simulink model "CONTROL_SYSTEM_V3_k"  (R2024a)
settings: Solver=ode1  StartTime=0.0  StopTime=inf  FixedStep=0.01  RelTol=1e-5
values from neighbouring files (symbols this model uses):
  Beta1 = 3*Omega_o    (= 15)    [CONTROL_SYSTEM_VAR.m]
  Beta2 = 3*(Omega_o^2)    (= 75)    [CONTROL_SYSTEM_VAR.m]
  Beta3 = (Omega_o^3)    (= 125)    [CONTROL_SYSTEM_VAR.m]
  Desire_Max = 255    [CONTROL_SYSTEM_VAR.m]
  Desire_Min = 0    [CONTROL_SYSTEM_VAR.m]
  Direction_Pin = 1    [CONTROL_SYSTEM_VAR.m]
  EN_Pin = 0    [CONTROL_SYSTEM_VAR.m]
  J_aet = 0.0035    [CONTROL_SYSTEM_VAR.m]
  Kd = 2    [CONTROL_SYSTEM_VAR.m]
  Ki = 4    [CONTROL_SYSTEM_VAR.m]
  Kn = 0.1    [CONTROL_SYSTEM_VAR.m]
  Kp = 1.4    [CONTROL_SYSTEM_VAR.m]
  omga_c = 10    [CONTROL_SYSTEM_VAR.m]
  roa = 0.24    [CONTROL_SYSTEM_VAR.m]
undefined symbols (not defined in the file or in its folder): sigbuilder_block
libraries: arduinolib x30, simulink_extras x14, simulink x5, slpidlib x4, spsOnDelayLib x2, slctrl_autotuning x2, slctrl_adaptive x1
(part 4 of 4)

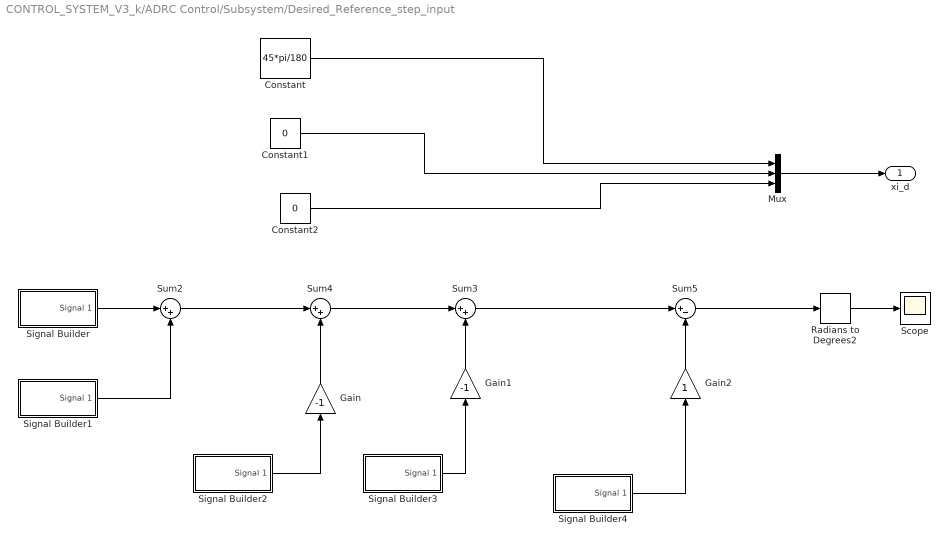
== system CONTROL_SYSTEM_V3_k/ADRC Control/Subsystem/Desired_Reference_step_input ==
  Constant : Constant  Value=45*pi/180
  Constant1 : Constant  Value=0
  Constant2 : Constant  Value=0
  Gain : Gain  Gain=-1
  Gain1 : Gain  Gain=-1
  Gain2 : Gain
  Mux : Mux  Inputs=3
  Radians to Degrees2 : simulink_extras/Transformations/Radians to Degrees
  Scope : Scope
  Signal Builder : Subsystem  Tag=STV Subsys  LoadFcn=sigbuilder_block('load');  StartFcn=sigbuilder_block('start');  StopFcn=sigbuilder_block('stop');  ClipboardFcn=sigbuilder_block('clipboard');  mask(Sigbuilder block){tuvar=[0:10]}
      mask help: Create and generate interchangeable groups of signals whose waveforms are piecewise linear.
      mask init:
      | if ~strcmp(get_param(bdroot(gcbh),'SimulationStatus'),'stopped') tuvar = sigbuilder_block('maskInit'); end
      settings: CopyFcn=sigbuilder_block('copy');  DeleteFcn=sigbuilder_block('delete');  ModelCloseFcn=sigbuilder_block('modelClose');  PreSaveFcn=sigbuilder_block('preSave');  PauseFcn=sigbuilder_block('pause')  ContinueFcn=sigbuilder_block('continue')  NameChangeFcn=sigbuilder_block('namechange');  OpenFcn=sigbuilder_block('open',[437.25 117.75 550.5 394.5 ]);  CloseFcn=sigbuilder_block('close');
      mask Display: plot(0, 0, 100, 100,[2, 2, 32, 32, 2], [68, 8, 8, 68, 68],[32, 2], [38, 38], [32, 19, 2],[53, 60, 44], [32, 17, 17, 2],[16, 16, 31, 31]);txt = getActiveGroup(gcbh);text(2, 100, txt,'verticalAlignment', 'top');
  Signal Builder1 : Subsystem  Tag=STV Subsys  LoadFcn=sigbuilder_block('load');  StartFcn=sigbuilder_block('start');  StopFcn=sigbuilder_block('stop');  ClipboardFcn=sigbuilder_block('clipboard');  mask(Sigbuilder block){tuvar=[0:10]}
      mask help: Create and generate interchangeable groups of signals whose waveforms are piecewise linear.
      mask init:
      | if ~strcmp(get_param(bdroot(gcbh),'SimulationStatus'),'stopped') tuvar = sigbuilder_block('maskInit'); end
      settings: CopyFcn=sigbuilder_block('copy');  DeleteFcn=sigbuilder_block('delete');  ModelCloseFcn=sigbuilder_block('modelClose');  PreSaveFcn=sigbuilder_block('preSave');  PauseFcn=sigbuilder_block('pause')  ContinueFcn=sigbuilder_block('continue')  NameChangeFcn=sigbuilder_block('namechange');  OpenFcn=sigbuilder_block('open',[153 72 550.2 394.8 ]);  CloseFcn=sigbuilder_block('close');
      mask Display: plot(0, 0, 100, 100,[2, 2, 32, 32, 2], [68, 8, 8, 68, 68],[32, 2], [38, 38], [32, 19, 2],[53, 60, 44], [32, 17, 17, 2],[16, 16, 31, 31]);txt = getActiveGroup(gcbh);text(2, 100, txt,'verticalAlignment', 'top');
  Signal Builder2 : Subsystem  Tag=STV Subsys  LoadFcn=sigbuilder_block('load');  StartFcn=sigbuilder_block('start');  StopFcn=sigbuilder_block('stop');  ClipboardFcn=sigbuilder_block('clipboard');  mask(Sigbuilder block){tuvar=[0:10]}
      mask help: Create and generate interchangeable groups of signals whose waveforms are piecewise linear.
      mask init:
      | if ~strcmp(get_param(bdroot(gcbh),'SimulationStatus'),'stopped') tuvar = sigbuilder_block('maskInit'); end
      settings: CopyFcn=sigbuilder_block('copy');  DeleteFcn=sigbuilder_block('delete');  ModelCloseFcn=sigbuilder_block('modelClose');  PreSaveFcn=sigbuilder_block('preSave');  PauseFcn=sigbuilder_block('pause')  ContinueFcn=sigbuilder_block('continue')  NameChangeFcn=sigbuilder_block('namechange');  OpenFcn=sigbuilder_block('open',[437.25 117.75 550.5 394.5 ]);  CloseFcn=sigbuilder_block('close');
      mask Display: plot(0, 0, 100, 100,[2, 2, 32, 32, 2], [68, 8, 8, 68, 68],[32, 2], [38, 38], [32, 19, 2],[53, 60, 44], [32, 17, 17, 2],[16, 16, 31, 31]);txt = getActiveGroup(gcbh);text(2, 100, txt,'verticalAlignment', 'top');
  Signal Builder3 : Subsystem  Tag=STV Subsys  LoadFcn=sigbuilder_block('load');  StartFcn=sigbuilder_block('start');  StopFcn=sigbuilder_block('stop');  ClipboardFcn=sigbuilder_block('clipboard');  mask(Sigbuilder block){tuvar=[0:10]}
      mask help: Create and generate interchangeable groups of signals whose waveforms are piecewise linear.
      mask init:
      | if ~strcmp(get_param(bdroot(gcbh),'SimulationStatus'),'stopped') tuvar = sigbuilder_block('maskInit'); end
      settings: CopyFcn=sigbuilder_block('copy');  DeleteFcn=sigbuilder_block('delete');  ModelCloseFcn=sigbuilder_block('modelClose');  PreSaveFcn=sigbuilder_block('preSave');  PauseFcn=sigbuilder_block('pause')  ContinueFcn=sigbuilder_block('continue')  NameChangeFcn=sigbuilder_block('namechange');  OpenFcn=sigbuilder_block('open',[437.25 117.75 550.5 394.5 ]);  CloseFcn=sigbuilder_block('close');
      mask Display: plot(0, 0, 100, 100,[2, 2, 32, 32, 2], [68, 8, 8, 68, 68],[32, 2], [38, 38], [32, 19, 2],[53, 60, 44], [32, 17, 17, 2],[16, 16, 31, 31]);txt = getActiveGroup(gcbh);text(2, 100, txt,'verticalAlignment', 'top');
  Signal Builder4 : Subsystem  Tag=STV Subsys  LoadFcn=sigbuilder_block('load');  StartFcn=sigbuilder_block('start');  StopFcn=sigbuilder_block('stop');  ClipboardFcn=sigbuilder_block('clipboard');  mask(Sigbuilder block){tuvar=[0:10]}
      mask help: Create and generate interchangeable groups of signals whose waveforms are piecewise linear.
      mask init:
      | if ~strcmp(get_param(bdroot(gcbh),'SimulationStatus'),'stopped') tuvar = sigbuilder_block('maskInit'); end
      settings: CopyFcn=sigbuilder_block('copy');  DeleteFcn=sigbuilder_block('delete');  ModelCloseFcn=sigbuilder_block('modelClose');  PreSaveFcn=sigbuilder_block('preSave');  PauseFcn=sigbuilder_block('pause')  ContinueFcn=sigbuilder_block('continue')  NameChangeFcn=sigbuilder_block('namechange');  OpenFcn=sigbuilder_block('open',[437.25 117.75 550.5 394.5 ]);  CloseFcn=sigbuilder_block('close');
      mask Display: plot(0, 0, 100, 100,[2, 2, 32, 32, 2], [68, 8, 8, 68, 68],[32, 2], [38, 38], [32, 19, 2],[53, 60, 44], [32, 17, 17, 2],[16, 16, 31, 31]);txt = getActiveGroup(gcbh);text(2, 100, txt,'verticalAlignment', 'top');
  Sum2 : Sum  Inputs=|++
  Sum3 : Sum  Inputs=|++
  Sum4 : Sum  Inputs=|++
  Sum5 : Sum  Inputs=|+-
  xi_d : Outport
  wires:
  Signal Builder/1(Signal 1) -> Sum2/1
  Signal Builder1/1(Signal 1) -> Sum2/2
  Sum2/1 -> Sum4/1
  Signal Builder2/1(Signal 1) -> Gain/1
  Gain/1 -> Sum4/2
  Sum4/1 -> Sum3/1
  Signal Builder3/1(Signal 1) -> Gain1/1
  Gain1/1 -> Sum3/2
  Sum3/1 -> Sum5/1
  Signal Builder4/1(Signal 1) -> Gain2/1
  Gain2/1 -> Sum5/2
  Sum5/1 -> Radians to Degrees2/1
  Radians to Degrees2/1 -> Scope/1
  Constant/1 -> Mux/1
  Mux/1 -> xi_d/1
  Constant1/1 -> Mux/2
  Constant2/1 -> Mux/3

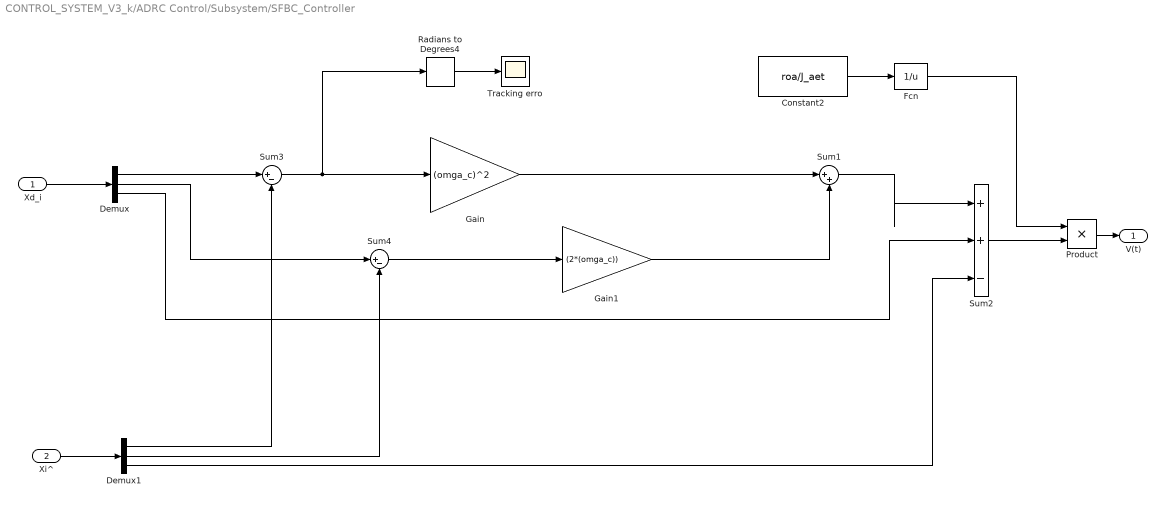
== system CONTROL_SYSTEM_V3_k/ADRC Control/Subsystem/SFBC_Controller ==
  Xd_i : Inport
  Xi^ : Inport  Port=2
  Constant2 : Constant  Value=roa/J_aet
  Demux : Demux  Outputs=3
  Demux1 : Demux  Outputs=3
  Fcn : Fcn  Expr=1/u
  Gain : Gain  Gain=(omga_c)^2
  Gain1 : Gain  Gain=(2*(omga_c))
  Product : Product  RndMeth=Zero
  Radians to Degrees4 : simulink_extras/Transformations/Radians to Degrees
  Sum1 : Sum  Inputs=|++
  Sum2 : Sum  Inputs=|++-
  Sum3 : Sum  Inputs=|+-
  Sum4 : Sum  Inputs=|+-
  Tracking erro : Scope
  V(t) : Outport
  wires:
  Gain/1 -> Sum1/1
  Gain1/1 -> Sum1/2
  Sum1/1 -> Sum2/1
  Constant2/1 -> Fcn/1
  Fcn/1 -> Product/1
  Sum2/1 -> Product/2
  Demux1/3 -> Sum2/3
  Product/1 -> V(t)/1
  Demux/3 -> Sum2/2
  Sum4/1 -> Gain1/1
  Xd_i/1 -> Demux/1
  Demux/1 -> Sum3/1
  Xi^/1 -> Demux1/1
  Demux1/1 -> Sum3/2
  Demux/2 -> Sum4/1
  Demux1/2 -> Sum4/2
  Sum3/1 -> Radians to Degrees4/1, Gain/1
  Radians to Degrees4/1 -> Tracking erro/1

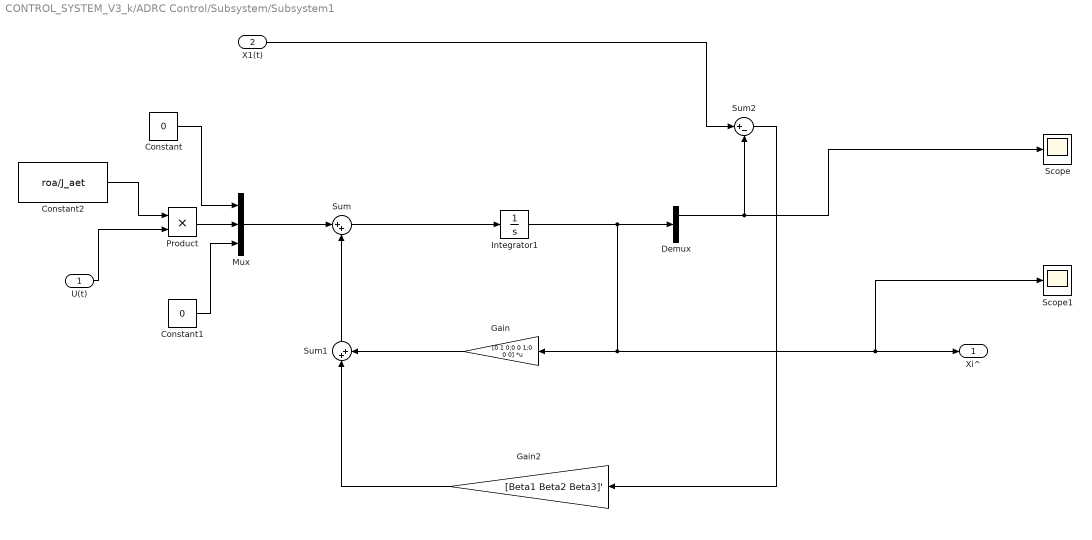
== system CONTROL_SYSTEM_V3_k/ADRC Control/Subsystem/Subsystem1 ==
  U(t) : Inport
  X1(t) : Inport  Port=2
  Constant : Constant  Value=0
  Constant1 : Constant  Value=0
  Constant2 : Constant  Value=roa/J_aet
  Demux : Demux  Outputs=3
  Gain : Gain  Gain=[0 1 0;0 0 1;0 0 0]  Multiplication=Matrix(K*u)
  Gain2 : Gain  Gain=[Beta1 Beta2 Beta3]'
  Integrator1 : Integrator  InitialCondition=[12*pi/180 0 0]'
  Mux : Mux  Inputs=3
  Product : Product  RndMeth=Zero
  Scope : Scope
  Scope1 : Scope
  Sum : Sum  Inputs=|++
  Sum1 : Sum  Inputs=|++
  Sum2 : Sum  Inputs=|+-
  Xi^ : Outport
  wires:
  Integrator1/1 -> Gain/1, Xi^/1, Scope1/1, Demux/1
  Sum/1 -> Integrator1/1
  Product/1 -> Mux/2
  Constant2/1 -> Product/1
  U(t)/1 -> Product/2
  Gain/1 -> Sum1/2
  Constant/1 -> Mux/1
  Constant1/1 -> Mux/3
  Mux/1 -> Sum/1
  Sum1/1 -> Sum/2
  Demux/1 -> Sum2/2, Scope/1
  X1(t)/1 -> Sum2/1
  Sum2/1 -> Gain2/1
  Gain2/1 -> Sum1/1

== system CONTROL_SYSTEM_V3_k/Subsystem5/ADRC Control1/Subsystem ==
  note: plot(Scope_e_ADRC.time, squeeze(Scope_e_ADRC.signals.values),Scope_e_AADRC.time, squeeze(Scope_e_AADRC.signals.values))
  note: kb=0.016
      | >> Ra=2.8
      | >> kt=0.016
      | >> J=4.0e-6
      | >> ktf=4.8e-3
      | >> kf=4e-4
      | >> theta_o=0.0349
      | >> ksp=0.0247
      | >> n=16.95
      | >> kpre=0.107
      | >> Vbat=0.24
      | omga_c=40
  note: Omega_o=120
      | >> Beta1=3*Omega_o
      | >> Beta2=3*(Omega_o^2)
      | >> Beta3=(Omega_o^3)
  X1(t) : Inport
  Contro_input (Voltages) : Scope
  Degrees to Radians1 : simulink_extras/Transformations/Degrees to Radians
  Desired signals_Sinewave : Subsystem
  Desired_Reference_step_input : Subsystem
  SFBC_Controller : Subsystem
  Subsystem1 : Subsystem
  V(t) : Outport
  wires:
  Degrees to Radians1/1 -> SFBC_Controller/1(Xd_i)
  SFBC_Controller/1(V(t)) -> V(t)/1, Contro_input (Voltages)/1, Subsystem1/1(U(t))
  Subsystem1/1(Xi^) -> SFBC_Controller/2(Xi^)
  X1(t)/1 -> Subsystem1/2(X1(t))
  Desired signals_Sinewave/1(xi_d) -> Degrees to Radians1/1
  Desired_Reference_step_input/1(xi_d) -> ?

== system CONTROL_SYSTEM_V3_k/ADRC Control/Subsystem/Desired_Reference_step_input/Signal Builder ==
  Demux : Demux  Tag=STV Demux  Outputs=1
      settings: DisplayOption=none
  FromWs : FromWorkspace  Tag=STV FromWs  VariableName=tuvar
      SigBuilderData=|
      | common.afterFinalStr = 'Extrapolate'
      | common.sampleTime = 0
      | dataSet.timeRange = [0 8]
      | dataSet.name = 'Group 1'
      | sbobj.Groups.Name = 'Group 1'
      | sbobj.Groups.Signals.Name = 'Signal 1'
      | sbobj.Groups.Signals.XData = [0 1 1 5 5 8]
      | sbobj.Groups.Signals.YData = [0 0 1.5 1.5 0 0]
      | sbobj.Groups.TimeRange = [0 8]
  Signal 1 : Outport  Tag=STV Outport
  wires:
  Demux/1 -> Signal 1/1
  FromWs/1 -> Demux/1

== system CONTROL_SYSTEM_V3_k/ADRC Control/Subsystem/Desired_Reference_step_input/Signal Builder1 ==
  Demux : Demux  Tag=STV Demux  Outputs=1
      settings: DisplayOption=none
  FromWs : FromWorkspace  Tag=STV FromWs  VariableName=tuvar
      SigBuilderData=|
      | common.afterFinalStr = 'Extrapolate'
      | common.sampleTime = 0
      | dataSet.timeRange = [0 14]
      | dataSet.name = 'Group 1'
      | sbobj.Groups.Name = 'Group 1'
      | sbobj.Groups.Signals.Name = 'Signal 1'
      | sbobj.Groups.Signals.XData = [0 9 9 13 13 14]
      | sbobj.Groups.Signals.YData = [0 0 1.5 1.5 1 1]
      | sbobj.Groups.TimeRange = [0 14]
  Signal 1 : Outport  Tag=STV Outport
  wires:
  Demux/1 -> Signal 1/1
  FromWs/1 -> Demux/1

== system CONTROL_SYSTEM_V3_k/ADRC Control/Subsystem/Desired_Reference_step_input/Signal Builder2 ==
  Demux : Demux  Tag=STV Demux  Outputs=1
      settings: DisplayOption=none
  FromWs : FromWorkspace  Tag=STV FromWs  VariableName=tuvar
      SigBuilderData=|
      | common.afterFinalStr = 'Extrapolate'
      | common.sampleTime = 0
      | dataSet.timeRange = [0 21]
      | dataSet.name = 'Group 1'
      | sbobj.Groups.Name = 'Group 1'
      | sbobj.Groups.Signals.Name = 'Signal 1'
      | sbobj.Groups.Signals.XData = [0 16.95 16.95 20 20 21]
      | sbobj.Groups.Signals.YData = [0 0 0.5 0.5 0 0]
      | sbobj.Groups.TimeRange = [0 21]
  Signal 1 : Outport  Tag=STV Outport
  wires:
  Demux/1 -> Signal 1/1
  FromWs/1 -> Demux/1

== system CONTROL_SYSTEM_V3_k/ADRC Control/Subsystem/Desired_Reference_step_input/Signal Builder3 ==
  Demux : Demux  Tag=STV Demux  Outputs=1
      settings: DisplayOption=none
  FromWs : FromWorkspace  Tag=STV FromWs  VariableName=tuvar
      SigBuilderData=|
      | common.afterFinalStr = 'Extrapolate'
      | common.sampleTime = 0
      | dataSet.timeRange = [0 25]
      | dataSet.name = 'Group 1'
      | sbobj.Groups.Name = 'Group 1'
      | sbobj.Groups.Signals.Name = 'Signal 1'
      | sbobj.Groups.Signals.XData = [0 20 20 21 21 25]
      | sbobj.Groups.Signals.YData = [0 0 0.5 0.5 0 0]
      | sbobj.Groups.TimeRange = [0 25]
  Signal 1 : Outport  Tag=STV Outport
  wires:
  Demux/1 -> Signal 1/1
  FromWs/1 -> Demux/1

== system CONTROL_SYSTEM_V3_k/ADRC Control/Subsystem/Desired_Reference_step_input/Signal Builder4 ==
  Demux : Demux  Tag=STV Demux  Outputs=1
      settings: DisplayOption=none
  FromWs : FromWorkspace  Tag=STV FromWs  VariableName=tuvar
      SigBuilderData=|
      | common.afterFinalStr = 'Extrapolate'
      | common.sampleTime = 0
      | dataSet.timeRange = [0 25]
      | dataSet.name = 'Group 1'
      | sbobj.Groups.Name = 'Group 1'
      | sbobj.Groups.Signals.Name = 'Signal 1'
      | sbobj.Groups.Signals.XData = [0 21 21 25]
      | sbobj.Groups.Signals.YData = [0 0 1 1]
      | sbobj.Groups.TimeRange = [0 25]
  Signal 1 : Outport  Tag=STV Outport
  wires:
  Demux/1 -> Signal 1/1
  FromWs/1 -> Demux/1

== system CONTROL_SYSTEM_V3_k/Subsystem5/ADRC Control1/Subsystem/Desired signals_Sinewave ==
  Clock : Clock
  Clock1 : Clock
  Clock2 : Clock
  Fcn1 : Fcn  Expr=10*sin(2*u)+10+7
  Fcn2 : Fcn  Expr=10*2*cos(2*u)
  Fcn3 : Fcn  Expr=-10*2*2*sin(2*u)
  Mux : Mux  Inputs=3
  xi_d : Outport
  wires:
  Clock/1 -> Fcn1/1
  Clock1/1 -> Fcn2/1
  Clock2/1 -> Fcn3/1
  Fcn1/1 -> Mux/1
  Fcn2/1 -> Mux/2
  Fcn3/1 -> Mux/3
  Mux/1 -> xi_d/1

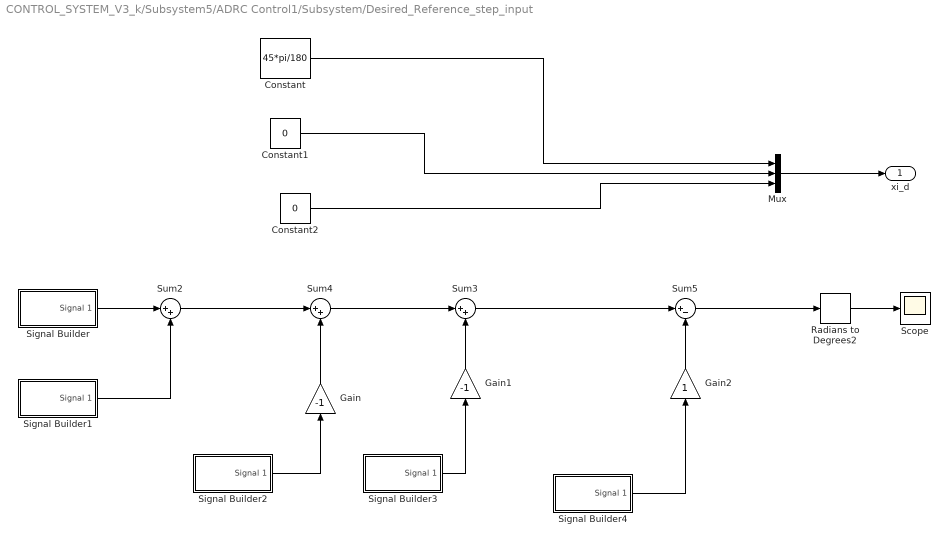
== system CONTROL_SYSTEM_V3_k/Subsystem5/ADRC Control1/Subsystem/Desired_Reference_step_input ==
  Constant : Constant  Value=45*pi/180
  Constant1 : Constant  Value=0
  Constant2 : Constant  Value=0
  Gain : Gain  Gain=-1
  Gain1 : Gain  Gain=-1
  Gain2 : Gain
  Mux : Mux  Inputs=3
  Radians to Degrees2 : simulink_extras/Transformations/Radians to Degrees
  Scope : Scope
  Signal Builder : Subsystem  Tag=STV Subsys  LoadFcn=sigbuilder_block('load');  StartFcn=sigbuilder_block('start');  StopFcn=sigbuilder_block('stop');  ClipboardFcn=sigbuilder_block('clipboard');  mask(Sigbuilder block){tuvar=[0:10]}
      mask help: Create and generate interchangeable groups of signals whose waveforms are piecewise linear.
      mask init:
      | if ~strcmp(get_param(bdroot(gcbh),'SimulationStatus'),'stopped') tuvar = sigbuilder_block('maskInit'); end
      settings: CopyFcn=sigbuilder_block('copy');  DeleteFcn=sigbuilder_block('delete');  ModelCloseFcn=sigbuilder_block('modelClose');  PreSaveFcn=sigbuilder_block('preSave');  PauseFcn=sigbuilder_block('pause')  ContinueFcn=sigbuilder_block('continue')  NameChangeFcn=sigbuilder_block('namechange');  OpenFcn=sigbuilder_block('open',[437.25 117.75 550.5 394.5 ]);  CloseFcn=sigbuilder_block('close');
      mask Display: plot(0, 0, 100, 100,[2, 2, 32, 32, 2], [68, 8, 8, 68, 68],[32, 2], [38, 38], [32, 19, 2],[53, 60, 44], [32, 17, 17, 2],[16, 16, 31, 31]);txt = getActiveGroup(gcbh);text(2, 100, txt,'verticalAlignment', 'top');
  Signal Builder1 : Subsystem  Tag=STV Subsys  LoadFcn=sigbuilder_block('load');  StartFcn=sigbuilder_block('start');  StopFcn=sigbuilder_block('stop');  ClipboardFcn=sigbuilder_block('clipboard');  mask(Sigbuilder block){tuvar=[0:10]}
      mask help: Create and generate interchangeable groups of signals whose waveforms are piecewise linear.
      mask init:
      | if ~strcmp(get_param(bdroot(gcbh),'SimulationStatus'),'stopped') tuvar = sigbuilder_block('maskInit'); end
      settings: CopyFcn=sigbuilder_block('copy');  DeleteFcn=sigbuilder_block('delete');  ModelCloseFcn=sigbuilder_block('modelClose');  PreSaveFcn=sigbuilder_block('preSave');  PauseFcn=sigbuilder_block('pause')  ContinueFcn=sigbuilder_block('continue')  NameChangeFcn=sigbuilder_block('namechange');  OpenFcn=sigbuilder_block('open',[153 72 550.2 394.8 ]);  CloseFcn=sigbuilder_block('close');
      mask Display: plot(0, 0, 100, 100,[2, 2, 32, 32, 2], [68, 8, 8, 68, 68],[32, 2], [38, 38], [32, 19, 2],[53, 60, 44], [32, 17, 17, 2],[16, 16, 31, 31]);txt = getActiveGroup(gcbh);text(2, 100, txt,'verticalAlignment', 'top');
  Signal Builder2 : Subsystem  Tag=STV Subsys  LoadFcn=sigbuilder_block('load');  StartFcn=sigbuilder_block('start');  StopFcn=sigbuilder_block('stop');  ClipboardFcn=sigbuilder_block('clipboard');  mask(Sigbuilder block){tuvar=[0:10]}
      mask help: Create and generate interchangeable groups of signals whose waveforms are piecewise linear.
      mask init:
      | if ~strcmp(get_param(bdroot(gcbh),'SimulationStatus'),'stopped') tuvar = sigbuilder_block('maskInit'); end
      settings: CopyFcn=sigbuilder_block('copy');  DeleteFcn=sigbuilder_block('delete');  ModelCloseFcn=sigbuilder_block('modelClose');  PreSaveFcn=sigbuilder_block('preSave');  PauseFcn=sigbuilder_block('pause')  ContinueFcn=sigbuilder_block('continue')  NameChangeFcn=sigbuilder_block('namechange');  OpenFcn=sigbuilder_block('open',[437.25 117.75 550.5 394.5 ]);  CloseFcn=sigbuilder_block('close');
      mask Display: plot(0, 0, 100, 100,[2, 2, 32, 32, 2], [68, 8, 8, 68, 68],[32, 2], [38, 38], [32, 19, 2],[53, 60, 44], [32, 17, 17, 2],[16, 16, 31, 31]);txt = getActiveGroup(gcbh);text(2, 100, txt,'verticalAlignment', 'top');
  Signal Builder3 : Subsystem  Tag=STV Subsys  LoadFcn=sigbuilder_block('load');  StartFcn=sigbuilder_block('start');  StopFcn=sigbuilder_block('stop');  ClipboardFcn=sigbuilder_block('clipboard');  mask(Sigbuilder block){tuvar=[0:10]}
      mask help: Create and generate interchangeable groups of signals whose waveforms are piecewise linear.
      mask init:
      | if ~strcmp(get_param(bdroot(gcbh),'SimulationStatus'),'stopped') tuvar = sigbuilder_block('maskInit'); end
      settings: CopyFcn=sigbuilder_block('copy');  DeleteFcn=sigbuilder_block('delete');  ModelCloseFcn=sigbuilder_block('modelClose');  PreSaveFcn=sigbuilder_block('preSave');  PauseFcn=sigbuilder_block('pause')  ContinueFcn=sigbuilder_block('continue')  NameChangeFcn=sigbuilder_block('namechange');  OpenFcn=sigbuilder_block('open',[437.25 117.75 550.5 394.5 ]);  CloseFcn=sigbuilder_block('close');
      mask Display: plot(0, 0, 100, 100,[2, 2, 32, 32, 2], [68, 8, 8, 68, 68],[32, 2], [38, 38], [32, 19, 2],[53, 60, 44], [32, 17, 17, 2],[16, 16, 31, 31]);txt = getActiveGroup(gcbh);text(2, 100, txt,'verticalAlignment', 'top');
  Signal Builder4 : Subsystem  Tag=STV Subsys  LoadFcn=sigbuilder_block('load');  StartFcn=sigbuilder_block('start');  StopFcn=sigbuilder_block('stop');  ClipboardFcn=sigbuilder_block('clipboard');  mask(Sigbuilder block){tuvar=[0:10]}
      mask help: Create and generate interchangeable groups of signals whose waveforms are piecewise linear.
      mask init:
      | if ~strcmp(get_param(bdroot(gcbh),'SimulationStatus'),'stopped') tuvar = sigbuilder_block('maskInit'); end
      settings: CopyFcn=sigbuilder_block('copy');  DeleteFcn=sigbuilder_block('delete');  ModelCloseFcn=sigbuilder_block('modelClose');  PreSaveFcn=sigbuilder_block('preSave');  PauseFcn=sigbuilder_block('pause')  ContinueFcn=sigbuilder_block('continue')  NameChangeFcn=sigbuilder_block('namechange');  OpenFcn=sigbuilder_block('open',[437.25 117.75 550.5 394.5 ]);  CloseFcn=sigbuilder_block('close');
      mask Display: plot(0, 0, 100, 100,[2, 2, 32, 32, 2], [68, 8, 8, 68, 68],[32, 2], [38, 38], [32, 19, 2],[53, 60, 44], [32, 17, 17, 2],[16, 16, 31, 31]);txt = getActiveGroup(gcbh);text(2, 100, txt,'verticalAlignment', 'top');
  Sum2 : Sum  Inputs=|++
  Sum3 : Sum  Inputs=|++
  Sum4 : Sum  Inputs=|++
  Sum5 : Sum  Inputs=|+-
  xi_d : Outport
  wires:
  Signal Builder/1(Signal 1) -> Sum2/1
  Signal Builder1/1(Signal 1) -> Sum2/2
  Sum2/1 -> Sum4/1
  Signal Builder2/1(Signal 1) -> Gain/1
  Gain/1 -> Sum4/2
  Sum4/1 -> Sum3/1
  Signal Builder3/1(Signal 1) -> Gain1/1
  Gain1/1 -> Sum3/2
  Sum3/1 -> Sum5/1
  Signal Builder4/1(Signal 1) -> Gain2/1
  Gain2/1 -> Sum5/2
  Sum5/1 -> Radians to Degrees2/1
  Radians to Degrees2/1 -> Scope/1
  Constant/1 -> Mux/1
  Mux/1 -> xi_d/1
  Constant1/1 -> Mux/2
  Constant2/1 -> Mux/3

== system CONTROL_SYSTEM_V3_k/Subsystem5/ADRC Control1/Subsystem/SFBC_Controller ==
  Xd_i : Inport
  Xi^ : Inport  Port=2
  Constant2 : Constant  Value=roa/J_aet
  Demux : Demux  Outputs=3
  Demux1 : Demux  Outputs=3
  Fcn : Fcn  Expr=1/u
  Gain : Gain  Gain=(omga_c)^2
  Gain1 : Gain  Gain=(2*(omga_c))
  Product : Product  RndMeth=Zero
  Radians to Degrees4 : simulink_extras/Transformations/Radians to Degrees
  Sum1 : Sum  Inputs=|++
  Sum2 : Sum  Inputs=|++-
  Sum3 : Sum  Inputs=|+-
  Sum4 : Sum  Inputs=|+-
  Tracking erro : Scope
  V(t) : Outport
  wires:
  Gain/1 -> Sum1/1
  Gain1/1 -> Sum1/2
  Sum1/1 -> Sum2/1
  Constant2/1 -> Fcn/1
  Fcn/1 -> Product/1
  Sum2/1 -> Product/2
  Demux1/3 -> Sum2/3
  Product/1 -> V(t)/1
  Demux/3 -> Sum2/2
  Sum4/1 -> Gain1/1
  Xd_i/1 -> Demux/1
  Demux/1 -> Sum3/1
  Xi^/1 -> Demux1/1
  Demux1/1 -> Sum3/2
  Demux/2 -> Sum4/1
  Demux1/2 -> Sum4/2
  Sum3/1 -> Radians to Degrees4/1, Gain/1
  Radians to Degrees4/1 -> Tracking erro/1

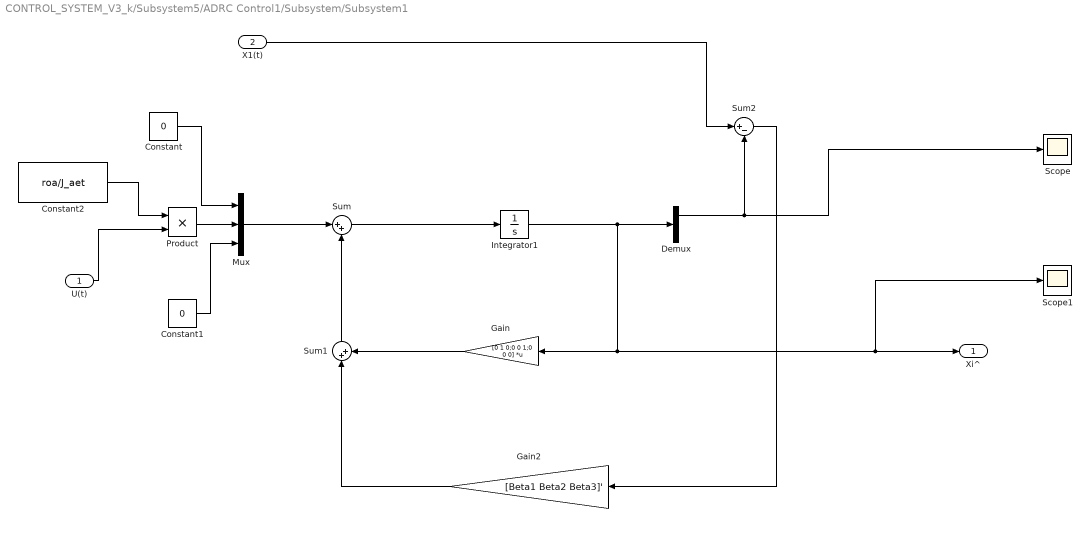
== system CONTROL_SYSTEM_V3_k/Subsystem5/ADRC Control1/Subsystem/Subsystem1 ==
  U(t) : Inport
  X1(t) : Inport  Port=2
  Constant : Constant  Value=0
  Constant1 : Constant  Value=0
  Constant2 : Constant  Value=roa/J_aet
  Demux : Demux  Outputs=3
  Gain : Gain  Gain=[0 1 0;0 0 1;0 0 0]  Multiplication=Matrix(K*u)
  Gain2 : Gain  Gain=[Beta1 Beta2 Beta3]'
  Integrator1 : Integrator  InitialCondition=[12*pi/180 0 0]'
  Mux : Mux  Inputs=3
  Product : Product  RndMeth=Zero
  Scope : Scope
  Scope1 : Scope
  Sum : Sum  Inputs=|++
  Sum1 : Sum  Inputs=|++
  Sum2 : Sum  Inputs=|+-
  Xi^ : Outport
  wires:
  Integrator1/1 -> Gain/1, Xi^/1, Scope1/1, Demux/1
  Sum/1 -> Integrator1/1
  Product/1 -> Mux/2
  Constant2/1 -> Product/1
  U(t)/1 -> Product/2
  Gain/1 -> Sum1/2
  Constant/1 -> Mux/1
  Constant1/1 -> Mux/3
  Mux/1 -> Sum/1
  Sum1/1 -> Sum/2
  Demux/1 -> Sum2/2, Scope/1
  X1(t)/1 -> Sum2/1
  Sum2/1 -> Gain2/1
  Gain2/1 -> Sum1/1

== system CONTROL_SYSTEM_V3_k/Subsystem5/ADRC Control1/Subsystem/Desired_Reference_step_input/Signal Builder ==
  Demux : Demux  Tag=STV Demux  Outputs=1
      settings: DisplayOption=none
  FromWs : FromWorkspace  Tag=STV FromWs  VariableName=tuvar
      SigBuilderData=|
      | common.afterFinalStr = 'Extrapolate'
      | common.sampleTime = 0
      | dataSet.timeRange = [0 8]
      | dataSet.name = 'Group 1'
      | sbobj.Groups.Name = 'Group 1'
      | sbobj.Groups.Signals.Name = 'Signal 1'
      | sbobj.Groups.Signals.XData = [0 1 1 5 5 8]
      | sbobj.Groups.Signals.YData = [0 0 1.5 1.5 0 0]
      | sbobj.Groups.TimeRange = [0 8]
  Signal 1 : Outport  Tag=STV Outport
  wires:
  Demux/1 -> Signal 1/1
  FromWs/1 -> Demux/1

== system CONTROL_SYSTEM_V3_k/Subsystem5/ADRC Control1/Subsystem/Desired_Reference_step_input/Signal Builder1 ==
  Demux : Demux  Tag=STV Demux  Outputs=1
      settings: DisplayOption=none
  FromWs : FromWorkspace  Tag=STV FromWs  VariableName=tuvar
      SigBuilderData=|
      | common.afterFinalStr = 'Extrapolate'
      | common.sampleTime = 0
      | dataSet.timeRange = [0 14]
      | dataSet.name = 'Group 1'
      | sbobj.Groups.Name = 'Group 1'
      | sbobj.Groups.Signals.Name = 'Signal 1'
      | sbobj.Groups.Signals.XData = [0 9 9 13 13 14]
      | sbobj.Groups.Signals.YData = [0 0 1.5 1.5 1 1]
      | sbobj.Groups.TimeRange = [0 14]
  Signal 1 : Outport  Tag=STV Outport
  wires:
  Demux/1 -> Signal 1/1
  FromWs/1 -> Demux/1

== system CONTROL_SYSTEM_V3_k/Subsystem5/ADRC Control1/Subsystem/Desired_Reference_step_input/Signal Builder2 ==
  Demux : Demux  Tag=STV Demux  Outputs=1
      settings: DisplayOption=none
  FromWs : FromWorkspace  Tag=STV FromWs  VariableName=tuvar
      SigBuilderData=|
      | common.afterFinalStr = 'Extrapolate'
      | common.sampleTime = 0
      | dataSet.timeRange = [0 21]
      | dataSet.name = 'Group 1'
      | sbobj.Groups.Name = 'Group 1'
      | sbobj.Groups.Signals.Name = 'Signal 1'
      | sbobj.Groups.Signals.XData = [0 16.95 16.95 20 20 21]
      | sbobj.Groups.Signals.YData = [0 0 0.5 0.5 0 0]
      | sbobj.Groups.TimeRange = [0 21]
  Signal 1 : Outport  Tag=STV Outport
  wires:
  Demux/1 -> Signal 1/1
  FromWs/1 -> Demux/1

== system CONTROL_SYSTEM_V3_k/Subsystem5/ADRC Control1/Subsystem/Desired_Reference_step_input/Signal Builder3 ==
  Demux : Demux  Tag=STV Demux  Outputs=1
      settings: DisplayOption=none
  FromWs : FromWorkspace  Tag=STV FromWs  VariableName=tuvar
      SigBuilderData=|
      | common.afterFinalStr = 'Extrapolate'
      | common.sampleTime = 0
      | dataSet.timeRange = [0 25]
      | dataSet.name = 'Group 1'
      | sbobj.Groups.Name = 'Group 1'
      | sbobj.Groups.Signals.Name = 'Signal 1'
      | sbobj.Groups.Signals.XData = [0 20 20 21 21 25]
      | sbobj.Groups.Signals.YData = [0 0 0.5 0.5 0 0]
      | sbobj.Groups.TimeRange = [0 25]
  Signal 1 : Outport  Tag=STV Outport
  wires:
  Demux/1 -> Signal 1/1
  FromWs/1 -> Demux/1

== system CONTROL_SYSTEM_V3_k/Subsystem5/ADRC Control1/Subsystem/Desired_Reference_step_input/Signal Builder4 ==
  Demux : Demux  Tag=STV Demux  Outputs=1
      settings: DisplayOption=none
  FromWs : FromWorkspace  Tag=STV FromWs  VariableName=tuvar
      SigBuilderData=|
      | common.afterFinalStr = 'Extrapolate'
      | common.sampleTime = 0
      | dataSet.timeRange = [0 25]
      | dataSet.name = 'Group 1'
      | sbobj.Groups.Name = 'Group 1'
      | sbobj.Groups.Signals.Name = 'Signal 1'
      | sbobj.Groups.Signals.XData = [0 21 21 25]
      | sbobj.Groups.Signals.YData = [0 0 1 1]
      | sbobj.Groups.TimeRange = [0 25]
  Signal 1 : Outport  Tag=STV Outport
  wires:
  Demux/1 -> Signal 1/1
  FromWs/1 -> Demux/1

== matlab function CONTROL_SYSTEM_V3_k/Subsystem5/Foot Pedal Calibration1 ==
  settings: updateMethod=DISCRETE
  data: PedalRange input; FP_maxVal output; FP_minVal output
function [FP_maxVal, FP_minVal] = FootPadel_Range(PedalRange)
    % Define a function FootPadel_Range that accepts a pedal position input (PedalRange)
    % and outputs the maximum and minimum values of the pedal position observed so far.
    
    % persistent variables to store maximum and minimum pedal values
    persistent maxSet minSet;
    
    % Initialize maxSet if it hasn't been set yet.
    if isempty(maxSet)
        maxSet = -1;  % Start with a value lower than the minimum possible PedalRange
    end
    
    % Initialize minSet if it hasn't been set yet.
    if isempty(minSet)
        minSet = 5;  % Start with a value higher than the maximum possible PedalRange
    end
    
    % Update maxSet if the current PedalRange is greater than the previous maxSet.
    if PedalRange > maxSet
        maxSet = PedalRange;
    end
    
    % Update minSet if the current PedalRange is less than the previous minSet.
    if PedalRange < minSet
        minSet = PedalRange;
    end
    
    % Assign the maximum and minimum values to the output variables.
    FP_maxVal = maxSet;
    FP_minVal = minSet;
end


% persistent maxSet minSet;: The persistent keyword is used to declare variables that retain their values between function calls. This is crucial for keeping track of the maximum and minimum pedal positions as the function is called multiple times.

% if isempty(maxSet) ... if isempty(minSet): These conditions ensure that the persistent variables are initialized only once, the first time the function is called.

% maxSet = PedalRange; minSet = PedalRange;: The maximum and minimum values are updated whenever a new extreme is found.

% FP_maxVal, FP_minVal: These output variables store the maximum and minimum pedal values, which are returned to the caller.

== matlab function CONTROL_SYSTEM_V3_k/Subsystem5/Throttle Body Callibration1 ==
  settings: updateMethod=DISCRETE
  data: TB_Range input; TB_maxVal output; TB_minVal output
function [TB_maxVal, TB_minVal] = ThrottleBody_Range(TB_Range)
    % Define a function ThrottleBody_Range that accepts a throttle body position input (TB_Range)
    % and outputs the maximum and minimum values of the throttle position observed so far.
    
    % Persistent variables to store maximum and minimum throttle body values
    persistent TB_maxSet TB_minSet;
    
    % Initialize TB_maxSet if it hasn't been set yet.
    if isempty(TB_maxSet)
        TB_maxSet = -1;  % Start with a value lower than the minimum possible TB_Range
    end
    
    % Initialize TB_minSet if it hasn't been set yet.
    if isempty(TB_minSet)
        TB_minSet = 5;  % Start with a value higher than the maximum possible TB_Range
    end
    
    % Update TB_maxSet if the current TB_Range is greater than the previous TB_maxSet.
    if TB_Range > TB_maxSet
        TB_maxSet = TB_Range;
    end
    
    % Update TB_minSet if the current TB_Range is less than the previous TB_minSet.
    if TB_Range < TB_minSet
        TB_minSet = TB_Range;
    end
    
    % Assign the maximum and minimum values to the output variables.
    TB_maxVal = TB_maxSet;
    TB_minVal = TB_minSet;
end

% persistent TB_maxSet TB_minSet: These persistent variables store the maximum and minimum throttle body positions. They retain their values across multiple calls to the function, allowing the function to keep track of the extremes over time.

% TB_maxSet = -1; TB_minSet = 5: These initial values are set to ensure that the first input will properly update the maximum and minimum values.

% TB_maxVal = TB_maxSet; TB_minVal = TB_minSet: These output variables return the current maximum and minimum throttle body values.

== matlab function CONTROL_SYSTEM_V3_k/Subsystem1/MATLAB Function ==
  data: Pedal_Val input; Desire_Val output
function Desire_Val = fcn(Pedal_Val)

persistent Previous_Val Set_Val
if isempty(Set_Val)
    Set_Val = 0;
end
if isempty(Previous_Val)
    Previous_Val = 0;
else
    Set_Val = abs(Previous_Val - Pedal_Val);
    Previous_Val = Pedal_Val;
end
Desire_Val = abs(Set_Val);
end

== matlab function CONTROL_SYSTEM_V3_k/Subsystem2/Throttle Body Callibration1 ==
  settings: updateMethod=DISCRETE
  data: TBRange input; TB_maxVal output; TB_minVal output
function [TB_maxVal, TB_minVal] = ThrottleBody_Range(TBRange)
    persistent TB_maxSet TB_minSet;
    if isempty(TB_maxSet)
        TB_maxSet = 0;
    end
    if isempty(TB_minSet)
        TB_minSet = 5; 
    end
    if TBRange > TB_maxSet
        TB_maxSet = TBRange;
    end
    if TBRange < TB_minSet
        TB_minSet = TBRange;
    end
    TB_maxVal = TB_maxSet;
    TB_minVal = TB_minSet;
end

== matlab function CONTROL_SYSTEM_V3_k/Subsystem6/Pedal Calibration1 ==
  settings: updateMethod=DISCRETE
  data: PedalRange input; FP_maxVal output; FP_minVal output
function [FP_maxVal, FP_minVal] = FootPadel_Range(PedalRange)
    persistent maxSet minSet;
    if isempty(maxSet)
        maxSet = -1;
    end
    if isempty(minSet)
        minSet = 5; 
    end
    if PedalRange > maxSet
        maxSet = PedalRange;
    end
    if PedalRange < minSet
        minSet = PedalRange;
    end
    FP_maxVal = maxSet;
    FP_minVal = minSet;
end

== matlab function CONTROL_SYSTEM_V3_k/Subsystem4/Pedal Calibration2 ==
  settings: updateMethod=DISCRETE
  data: PedalRange input; FP_maxVal output; FP_minVal output; Calibration_Input input
function [FP_maxVal, FP_minVal] = FootPadel_Range(PedalRange, Calibration_Input)
    persistent maxSet minSet;
    if isempty(maxSet)
        maxSet = 0;
    end
    if isempty(minSet)
        minSet = 5;
    end
    if PedalRange > maxSet
        maxSet = PedalRange;
    end
    if PedalRange < minSet
        minSet = PedalRange;
    end
    FP_maxVal = maxSet;
    FP_minVal = minSet;
    if Calibration_Input == 1
        maxSet = 0;
        minSet = 5;
    end
end

== matlab function CONTROL_SYSTEM_V3_k/Subsystem6/Throttle Body Callibration2 ==
  settings: updateMethod=DISCRETE
  data: TBRange input; TB_maxVal output; TB_minVal output
function [TB_maxVal, TB_minVal] = ThrottleBody_Range(TBRange)
    persistent TB_maxSet TB_minSet;
    if isempty(TB_maxSet)
        TB_maxSet = 0;
    end
    if isempty(TB_minSet)
        TB_minSet = 5; 
    end
    if TBRange > TB_maxSet
        TB_maxSet = TBRange;
    end
    if TBRange < TB_minSet
        TB_minSet = TBRange;
    end
    TB_maxVal = TB_maxSet;
    TB_minVal = TB_minSet;
end

== matlab function CONTROL_SYSTEM_V3_k/Subsystem4/Throttle Body Callibration1 ==
  settings: updateMethod=DISCRETE
  data: TBRange input; TB_maxVal output; TB_minVal output; Calibration_Input input
function [TB_maxVal, TB_minVal] = ThrottleBody_Range(TBRange, Calibration_Input)
    persistent TB_maxSet TB_minSet;
    if isempty(TB_maxSet)
        TB_maxSet = 0;
    end
    if isempty(TB_minSet)
        TB_minSet = 5;
    end
    if TBRange > TB_maxSet
        TB_maxSet = TBRange;
    end
    if TBRange < TB_minSet
        TB_minSet = TBRange;
    end
    TB_maxVal = TB_maxSet;
    TB_minVal = TB_minSet;
    if Calibration_Input == 1
        TB_maxSet = 0;
        TB_minSet = 5;
    end
end

== matlab function CONTROL_SYSTEM_V3_k/Foot Pedal Calibration ==
  settings: updateMethod=DISCRETE
  data: PedalRange input; FP_maxVal output; FP_minVal output
function [FP_maxVal, FP_minVal] = FootPadel_Range(PedalRange)
    % Define a function FootPadel_Range that accepts a pedal position input (PedalRange)
    % and outputs the maximum and minimum values of the pedal position observed so far.
    
    % persistent variables to store maximum and minimum pedal values
    persistent maxSet minSet;
    
    % Initialize maxSet if it hasn't been set yet.
    if isempty(maxSet)
        maxSet = -1;  % Start with a value lower than the minimum possible PedalRange
    end
    
    % Initialize minSet if it hasn't been set yet.
    if isempty(minSet)
        minSet = 5;  % Start with a value higher than the maximum possible PedalRange
    end
    
    % Update maxSet if the current PedalRange is greater than the previous maxSet.
    if PedalRange > maxSet
        maxSet = PedalRange;
    end
    
    % Update minSet if the current PedalRange is less than the previous minSet.
    if PedalRange < minSet
        minSet = PedalRange;
    end
    
    % Assign the maximum and minimum values to the output variables.
    FP_maxVal = maxSet;
    FP_minVal = minSet;
end


% persistent maxSet minSet;: The persistent keyword is used to declare variables that retain their values between function calls. This is crucial for keeping track of the maximum and minimum pedal positions as the function is called multiple times.

% if isempty(maxSet) ... if isempty(minSet): These conditions ensure that the persistent variables are initialized only once, the first time the function is called.

% maxSet = PedalRange; minSet = PedalRange;: The maximum and minimum values are updated whenever a new extreme is found.

% FP_maxVal, FP_minVal: These output variables store the maximum and minimum pedal values, which are returned to the caller.

== matlab function CONTROL_SYSTEM_V3_k/Throttle Body Callibration ==
  settings: updateMethod=DISCRETE
  data: TB_Range input; TB_maxVal output; TB_minVal output
function [TB_maxVal, TB_minVal] = ThrottleBody_Range(TB_Range)
    % Define a function ThrottleBody_Range that accepts a throttle body position input (TB_Range)
    % and outputs the maximum and minimum values of the throttle position observed so far.
    
    % Persistent variables to store maximum and minimum throttle body values
    persistent TB_maxSet TB_minSet;
    
    % Initialize TB_maxSet if it hasn't been set yet.
    if isempty(TB_maxSet)
        TB_maxSet = -1;  % Start with a value lower than the minimum possible TB_Range
    end
    
    % Initialize TB_minSet if it hasn't been set yet.
    if isempty(TB_minSet)
        TB_minSet = 5;  % Start with a value higher than the maximum possible TB_Range
    end
    
    % Update TB_maxSet if the current TB_Range is greater than the previous TB_maxSet.
    if TB_Range > TB_maxSet
        TB_maxSet = TB_Range;
    end
    
    % Update TB_minSet if the current TB_Range is less than the previous TB_minSet.
    if TB_Range < TB_minSet
        TB_minSet = TB_Range;
    end
    
    % Assign the maximum and minimum values to the output variables.
    TB_maxVal = TB_maxSet;
    TB_minVal = TB_minSet;
end

% persistent TB_maxSet TB_minSet: These persistent variables store the maximum and minimum throttle body positions. They retain their values across multiple calls to the function, allowing the function to keep track of the extremes over time.

% TB_maxSet = -1; TB_minSet = 5: These initial values are set to ensure that the first input will properly update the maximum and minimum values.

% TB_maxVal = TB_maxSet; TB_minVal = TB_minSet: These output variables return the current maximum and minimum throttle body values.
